simulink model "Key_signal_jump_abnormal_check"  (R2021a)
settings: configuration reference "ART_1G_IDS_Speedgoat" (kept outside this file)
libraries: simulink x1
settings Model: DataDictionary=Key_Signal_Jump_Abnormal_Check.sldd  Creator=xinrui  LastModifiedBy=xinrui
settings ConfigSetRef: SourceName=ART_1G_IDS_Speedgoat

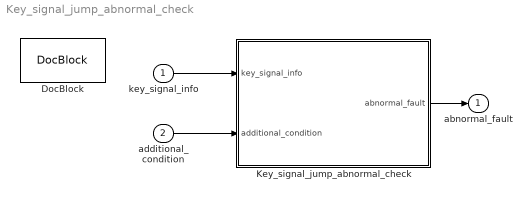
== system Key_signal_jump_abnormal_check ==
  "key_signal_info " : Inport  OutDataTypeStr=Bus: Key_Signal_Info  PortDimensions=1
  additional_condition : Inport  Port=2  OutDataTypeStr=Enum: Validation  PortDimensions=1
  DocBlock : simulink/Model-Wide Utilities/DocBlock  DocumentType=HTML  mask(DocBlock){}
      mask Display:
      | plot([.8 0 0 1 1 .8 .8 1],[1 1 0 0 .8 1 .8 .8]);
      | text(.5,.6,'CHANGELOG','horizontalalignment','center');
      | text(.95,.05,get_param(gcb,'DocumentType'),'verticalalignment','bottom','horizontalalignment','right');
  Key_signal_jump_abnormal_check : Stateflow chart  TreatAsAtomicUnit=on
  abnormal_fault : Outport  OutDataTypeStr=Enum: Validation  PortDimensions=1
  wires:
  "key_signal_info "/1 -> Key_signal_jump_abnormal_check/1(key_signal_info)
  Key_signal_jump_abnormal_check/1(abnormal_fault) -> abnormal_fault/1
  additional_condition/1 -> Key_signal_jump_abnormal_check/2(additional_condition)

== stateflow chart Key_signal_jump_abnormal_check/Key_signal_jump_abnormal_check ==
  settings: updateMethod=DISCRETE
  state key_signal_jump_abnormal_check %关键信号突变检测
    abnormal_condition = key_signal_info.jump_abnormal_tolerance < fabs(key_signal_info.original_value_current - key_signal_info.original_value_previous);
    is_normal = key_signal_info.recovery_check_times <= recovery_check_counter;
    need_observing = Validation.Invalid == abnormal_condition;
    is_abnormal = Validation.Valid == abnormal_condition && Validation.Valid == additional_condition;
    state normal %正常
      abnormal_fault = Validation.Invalid;
    state abnormal %异常
      abnormal_fault = Validation.Valid;
    state observation %观测
      recovery_check_counter++;
    normal %正常 -> abnormal %异常 : [is_abnormal]
    (default) -> normal %正常
    observation %观测 -> normal %正常 [order 1] : [is_normal]
    observation %观测 -> abnormal %异常 [order 2] : [is_abnormal]
    abnormal %异常 -> observation %观测 : [need_observing]{recovery_check_counter = 0}
  (default) -> key_signal_jump_abnormal_check %关键信号突变检测 : {recovery_check_counter = 0;}
  data: key_signal_info input Bus: Key_Signal_Info; additional_condition input Enum: Validation; abnormal_fault output Enum: Validation; is_abnormal local boolean; need_observing local boolean; is_normal local boolean; abnormal_condition local Enum: Validation; recovery_check_counter local uint32
